simulink model "VMC_Integration"  (R2024a)
settings: Solver=FixedStepDiscrete  StartTime=0.0  StopTime=10.0  FixedStep=0.005  RelTol=1e-3
undefined symbols (not defined in the file): Degree_To_Rad_Factor
libraries: simulink x24, slpidlib x5
(part 1 of 3)
settings Model: Creator=Technic  LastModifiedBy=Technic
settings SolverCC: ZeroCrossControl=EnableAll
settings OptimizationCC: DefaultParameterBehavior=Inlined  DefaultUnderspecifiedDataType=single  EnhancedBackFolding=on  PassReuseOutputArgsAs=Individual arguments  ZeroExternalMemoryAtStartup=off  ZeroInternalMemoryAtStartup=off  OptimizeBlockOrder=speed  DifferentSizesBufferReuse=on  OptimizationCustomize=off  EfficientTunableParamExpr=on
settings DebuggingCC: AlgebraicLoopMsg=error  BlockPriorityViolationMsg=error  SolverPrmCheckMsg=error  ParameterPrecisionLossMsg=none  ParamPrecisionLossAbsoluteDiffThreshold=1e-12  ParamPrecisionLossRelativeDiffThreshold=1e-10  ParameterTunabilityLossMsg=error  UnnecessaryDatatypeConvMsg=warning  StateNameClashWarn=warning  AllowedUnitSystems=SI,SI (extended)  AllowAutomaticUnitConversions=off
settings HardwareCC: ProdBitPerPointer=32  ProdBitPerSizeT=32  ProdBitPerPtrDiffT=32  ProdLargestAtomicInteger=Long  ProdLargestAtomicFloat=Double  ProdWordSize=32  ProdHWDeviceType=NXP->Cortex-M4
settings SFSimCC: MATLABDynamicMemAlloc=off
settings RTWCC: Description=Embedded Coder  SystemTargetFile=ert.tlc  GenCodeOnly=on  TemplateMakefile=ert_default_tmf  GenerateReport=on  LaunchReport=on
settings CodeAppCC: ForceParamTrailComments=on  IgnoreCustomStorageClasses=off  OperatorAnnotations=on  SimulinkDataObjDesc=on  SFDataObjDesc=on  InsertBlockDesc=on
settings ERTTargetCC: TargetLangStandard=C99 (ISO)  GenerateSampleERTMain=on  InlinedParameterPlacement=NonHierarchical  ERTCustomFileTemplate=example_file_process.tlc

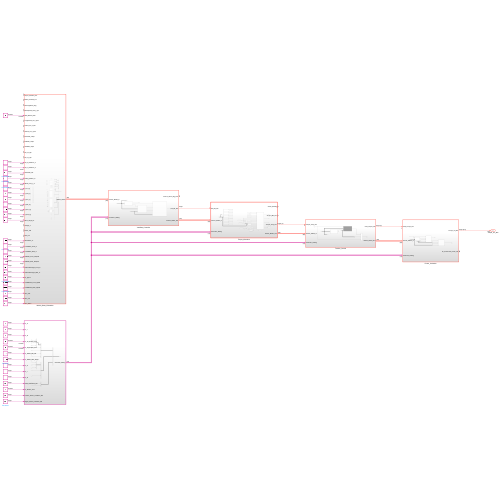
[thumbnail: Simulink's stored preview of the top-level diagram]
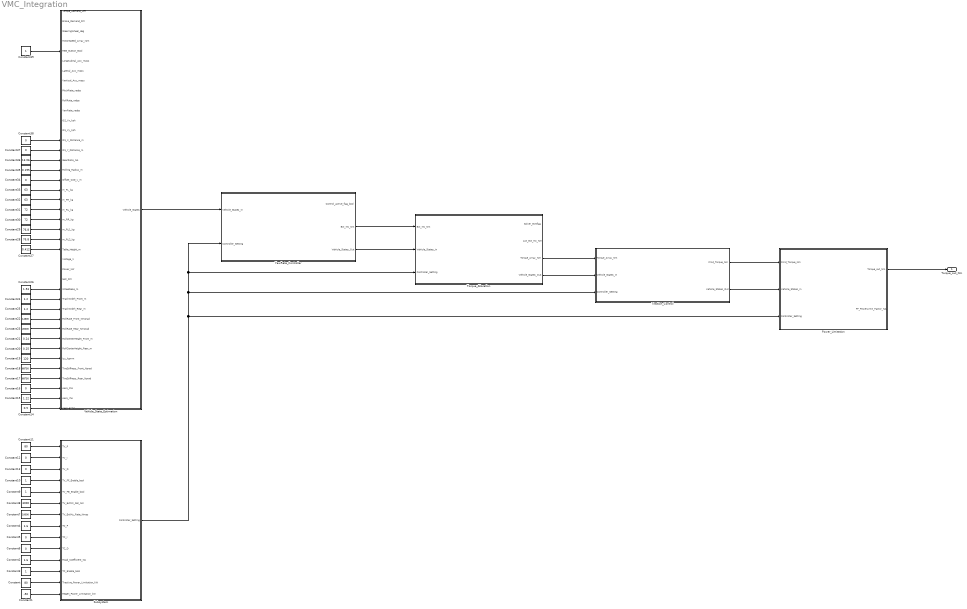
== system VMC_Integration ==
  Constant : Constant  Value=80  OutDataTypeStr=single
  Constant1 : Constant  Value=-50  OutDataTypeStr=single
  Constant{3,9..10,39} (4 alike) : Constant  OutDataTypeStr=boolean
  Constant11 : Constant  Value=80  OutDataTypeStr=single
  Constant{5..6,12..13,16,34,37..38} (8 alike) : Constant  Value=0  OutDataTypeStr=single
  Constant14 : Constant  Value=0.5  OutDataTypeStr=single
  Constant15 : Constant  Value=1.22  OutDataTypeStr=single
  Constant17 : Constant  Value=68750  OutDataTypeStr=single
  Constant18 : Constant  Value=68750  OutDataTypeStr=single
  Constant19 : Constant  Value=120  OutDataTypeStr=single
  Constant2 : Constant  Value=1.6  OutDataTypeStr=single
  Constant20 : Constant  Value=0.25  OutDataTypeStr=single
  Constant21 : Constant  Value=0.24  OutDataTypeStr=single
  Constant22 : Constant  Value=14600  OutDataTypeStr=single
  Constant23 : Constant  Value=45000  OutDataTypeStr=single
  Constant24 : Constant  Value=1.2  OutDataTypeStr=single
  Constant25 : Constant  Value=1.2  OutDataTypeStr=single
  Constant26 : Constant  Value=1.53  OutDataTypeStr=single
  Constant27 : Constant  Value=0.412  OutDataTypeStr=single
  Constant28 : Constant  Value=76.8  OutDataTypeStr=single
  Constant29 : Constant  Value=76.8  OutDataTypeStr=single
  Constant30 : Constant  Value=72  OutDataTypeStr=single
  Constant31 : Constant  Value=72  OutDataTypeStr=single
  Constant32 : Constant  Value=63  OutDataTypeStr=single
  Constant33 : Constant  Value=63  OutDataTypeStr=single
  Constant35 : Constant  Value=0.195  OutDataTypeStr=single
  Constant36 : Constant  Value=13.06  OutDataTypeStr=single
  Constant4 : Constant  Value=1.6  OutDataTypeStr=single
  Constant7 : Constant  Value=10000  OutDataTypeStr=single
  Constant8 : Constant  Value=3000  OutDataTypeStr=single
  Power_Limitation : Subsystem
  Subsystem : Subsystem
  Torque_Allocation : Subsystem  TreatAsAtomicUnit=on  RTWFcnName=Torque_Allocation
      settings: RTWSystemCode=Nonreusable function  RTWFcnNameOpts=User specified
  Traction_Control : Subsystem
  Vehicle_State_Estimation : Subsystem
  YawRate_Controller : Subsystem
  Torque_out_Nm : Outport
  wires:
  Vehicle_State_Estimation/1(Vehicle_States) -> YawRate_Controller/1(Vehicle_States_In)
  Subsystem/1(Controller_Setting) -> Torque_Allocation/3(Controller_Setting), YawRate_Controller/2(Controller_Setting), Traction_Control/3(Controller_Setting), Power_Limitation/3(Controller_Setting)
  YawRate_Controller/2(Ext_Mz_Nm) -> Torque_Allocation/1(Ext_Mz_Nm)
  YawRate_Controller/3(Vehicle_States_Out) -> Torque_Allocation/2(Vehicle_States_In)
  Torque_Allocation/3(Torque_Array_Nm) -> Traction_Control/1(Torque_Array_Nm)
  Traction_Control/2(Vehicle_States_Out) -> Power_Limitation/2(Vehicle_States_In)
  Traction_Control/1(Cmd_Torque_Nm) -> Power_Limitation/1(Cmd_Torque_Nm)
  Constant/1 -> Subsystem/13(Tractive_Power_Limitation_kW)
  Constant1/1 -> Subsystem/14(Regen_Power_Limitation_kW)
  Torque_Allocation/4(Vehicle_States_Out) -> Traction_Control/2(Vehicle_States_In)
  Power_Limitation/1(Torque_out_Nm) -> Torque_out_Nm/1
  Constant2/1 -> Subsystem/11(Road_Coefficient_NA)
  Constant3/1 -> Subsystem/12(TC_Enable_bool)
  Constant4/1 -> Subsystem/8(TC_P)
  Constant5/1 -> Subsystem/9(TC_I)
  Constant6/1 -> Subsystem/10(TC_D)
  Constant7/1 -> Subsystem/7(TV_ExtMz_Rate_Nmps)
  Constant8/1 -> Subsystem/6(TV_ExtMz_Sat_Nm)
  Constant9/1 -> Subsystem/5(TV_FB_Enable_bool)
  Constant10/1 -> Subsystem/4(TV_FF_Enable_bool)
  Constant11/1 -> Subsystem/1(TV_P)
  Constant12/1 -> Subsystem/2(TV_I)
  Constant13/1 -> Subsystem/3(TV_D)
  Constant14/1 -> Vehicle_State_Estimation/41(Aero_Ratio)
  Constant15/1 -> Vehicle_State_Estimation/40(Aero_rho)
  Constant16/1 -> Vehicle_State_Estimation/39(Aero_ClA)
  Constant17/1 -> Vehicle_State_Estimation/38(TireStiffness_Rear_Nprad)
  Constant18/1 -> Vehicle_State_Estimation/37(TireStiffness_Front_Nprad)
  Constant19/1 -> Vehicle_State_Estimation/36(Izz_kgmm)
  Constant20/1 -> Vehicle_State_Estimation/35(RollCenterHeight_Rear_m)
  Constant21/1 -> Vehicle_State_Estimation/34(RollCenterHeight_Front_m)
  Constant22/1 -> Vehicle_State_Estimation/32(RollRate_Front_Nmprad)
  Constant23/1 -> Vehicle_State_Estimation/33(RollRate_Rear_Nmprad)
  Constant24/1 -> Vehicle_State_Estimation/30(TrackWidth_Front_m)
  Constant25/1 -> Vehicle_State_Estimation/31(TrackWidth_Rear_m)
  Constant26/1 -> Vehicle_State_Estimation/29(Wheelbase_m)
  Constant27/1 -> Vehicle_State_Estimation/25(Table_Height_m)
  Constant28/1 -> Vehicle_State_Estimation/24(m_RL2_kg)
  Constant29/1 -> Vehicle_State_Estimation/23(m_RL1_kg)
  Constant30/1 -> Vehicle_State_Estimation/22(m_RR_kg)
  Constant31/1 -> Vehicle_State_Estimation/21(m_RL_kg)
  Constant32/1 -> Vehicle_State_Estimation/20(m_FR_kg)
  Constant33/1 -> Vehicle_State_Estimation/19(m_FL_kg)
  Constant34/1 -> Vehicle_State_Estimation/18(Offset_CoG_y_m)
  Constant35/1 -> Vehicle_State_Estimation/17(Rolling_Radius_m)
  Constant36/1 -> Vehicle_State_Estimation/16(GearRatio_NA)
  Constant37/1 -> Vehicle_State_Estimation/15(OS_Y_Distance_m)
  Constant38/1 -> Vehicle_State_Estimation/14(OS_X_Distance_m)
  Constant39/1 -> Vehicle_State_Estimation/5(REG_Button_Bool)

== system VMC_Integration/Power_Limitation ==
  Cmd_Torque_Nm : Inport
  Vehicle_States_In : Inport  Port=2
  Controller_Setting : Inport  Port=3
  Bus Selector : BusSelector  OutputSignals=Power_Limitation.Tractive_Power_Limitation_kW,Power_Limitation.Regen_Power_Limitation_kW
  Bus Selector1 : BusSelector  OutputSignals=Power_Limitation.Tractive_Power_Limitation_kW,Power_Limitation.Regen_Power_Limitation_kW
  Bus Selector2 : BusSelector  OutputSignals=Accumulator.Power_kW
  FeedForward_PowerLimit : MATLAB Function  TreatAsAtomicUnit=on
  MATLAB Function : MATLAB Function  TreatAsAtomicUnit=on
  Power_Estimation : Subsystem
  Torque_out_Nm : Outport
  FF_PowerLimit_Factor_NA : Outport  Port=2
  wires:
  Vehicle_States_In/1 -> Bus Selector2/1, Power_Estimation/2(Vehicle_States_In)
  Cmd_Torque_Nm/1 -> Power_Estimation/1(Cmd_Torque_Nm), FeedForward_PowerLimit/1(Torque)
  Controller_Setting/1 -> Bus Selector1/1, Bus Selector/1
  Bus Selector/1 -> FeedForward_PowerLimit/3(Tractive_Limit_Power)  "<Tractive_Power_Limitation_kW>"
  Power_Estimation/1(Est_Power_kW) -> FeedForward_PowerLimit/2(Est_Power)
  Bus Selector/2 -> FeedForward_PowerLimit/4(Regen_Limit_Power)  "<Regen_Power_Limitation_kW>"
  FeedForward_PowerLimit/2(Torque_out) -> MATLAB Function/1(Torque)
  Bus Selector1/1 -> MATLAB Function/2(Tractive_Limit_Power)  "<Tractive_Power_Limitation_kW>"
  Bus Selector1/2 -> MATLAB Function/3(Regen_Limit_Power)  "<Regen_Power_Limitation_kW>"
  Bus Selector2/1 -> MATLAB Function/4(Act_Power)  "<Power_kW>"
  MATLAB Function/1(Torque_out) -> Torque_out_Nm/1
  FeedForward_PowerLimit/1(factor) -> FF_PowerLimit_Factor_NA/1

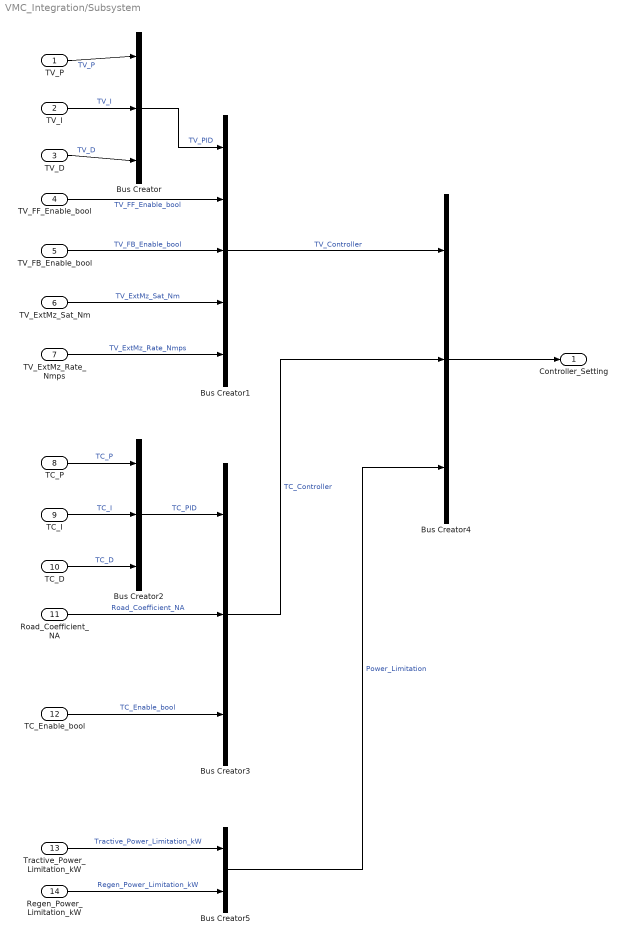
== system VMC_Integration/Subsystem ==
  TV_P : Inport
  TV_I : Inport  Port=2
  TV_D : Inport  Port=3
  TV_FF_Enable_bool : Inport  Port=4  OutDataTypeStr=boolean
  TV_FB_Enable_bool : Inport  Port=5  OutDataTypeStr=boolean
  TV_ExtMz_Sat_Nm : Inport  Port=6
  TV_ExtMz_Rate_Nmps : Inport  Port=7
  TC_P : Inport  Port=8
  TC_I : Inport  Port=9
  TC_D : Inport  Port=10
  Road_Coefficient_NA : Inport  Port=11
  TC_Enable_bool : Inport  Port=12
  Tractive_Power_Limitation_kW : Inport  Port=13
  Regen_Power_Limitation_kW : Inport  Port=14
  Bus Creator{,2..4} (4 alike) : BusCreator  Inputs=3
  Bus Creator1 : BusCreator  Inputs=5
  Bus Creator5 : BusCreator  Inputs=2
  Controller_Setting : Outport
  wires:
  TV_P/1 -> Bus Creator/1  "TV_P"
  TV_I/1 -> Bus Creator/2  "TV_I"
  TV_D/1 -> Bus Creator/3  "TV_D"
  Bus Creator/1 -> Bus Creator1/1  "TV_PID"
  TV_FF_Enable_bool/1 -> Bus Creator1/2  "TV_FF_Enable_bool"
  TV_FB_Enable_bool/1 -> Bus Creator1/3  "TV_FB_Enable_bool"
  TV_ExtMz_Sat_Nm/1 -> Bus Creator1/4  "TV_ExtMz_Sat_Nm"
  TV_ExtMz_Rate_Nmps/1 -> Bus Creator1/5  "TV_ExtMz_Rate_Nmps"
  TC_P/1 -> Bus Creator2/1  "TC_P"
  TC_I/1 -> Bus Creator2/2  "TC_I"
  TC_D/1 -> Bus Creator2/3  "TC_D"
  Bus Creator2/1 -> Bus Creator3/1  "TC_PID"
  Bus Creator1/1 -> Bus Creator4/1  "TV_Controller"
  Bus Creator3/1 -> Bus Creator4/2  "TC_Controller"
  Bus Creator4/1 -> Controller_Setting/1
  Road_Coefficient_NA/1 -> Bus Creator3/2  "Road_Coefficient_NA"
  TC_Enable_bool/1 -> Bus Creator3/3  "TC_Enable_bool"
  Bus Creator5/1 -> Bus Creator4/3  "Power_Limitation"
  Tractive_Power_Limitation_kW/1 -> Bus Creator5/1  "Tractive_Power_Limitation_kW"
  Regen_Power_Limitation_kW/1 -> Bus Creator5/2  "Regen_Power_Limitation_kW"

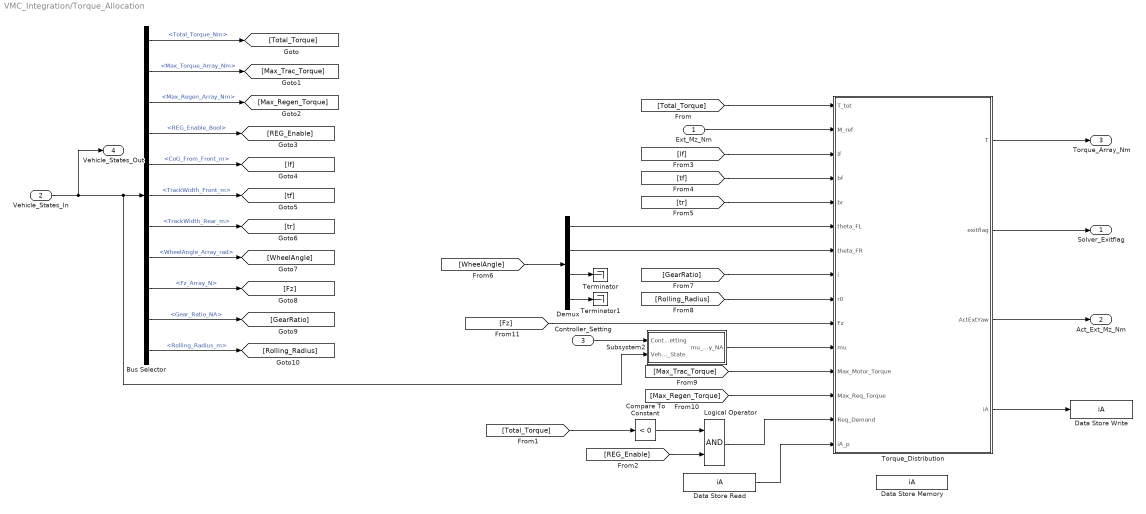
== system VMC_Integration/Torque_Allocation ==
  Ext_Mz_Nm : Inport
  Vehicle_States_In : Inport  Port=2
  Controller_Setting : Inport  Port=3
  Bus Selector : BusSelector  OutputSignals=Torque_Demand.Total_Torque_Nm,Torque_Demand.Max_Torque_Array_Nm,Torque_Demand.Max_Regen_Array_Nm,Torque_Demand.REG_Enable_Bool,Vehicle_Static_Parameter.CoG_From_Front_m,Vehicle_Static_Parameter.TrackWidth_Front_m,Vehicle_Static_Parameter.TrackWidth_Rear_m,WheelAngle.WheelAngle_Array_rad,Tire_Force.Fz_Array_N,Vehicle_Static_Parameter.Gear_Ratio_NA,Vehicle_Static_Parameter.Rolling_Radius_m
  Compare To Constant : simulink/Logic and Bit Operations/Compare To Constant  relop=<  const=0  OutDataTypeStr=boolean
  Data Store Memory : DataStoreMemory  DataStoreName=iA  WriteAfterWriteMsg=warning  InitialValue=[0,0,0,0,0,0,0,0]  ShowAdditionalParam=off  OutDataTypeStr=boolean
  Data Store Read : DataStoreRead  DataStoreName=iA  IndexOptions=Index vector (dialog)  Indices=1  OutputSizes=1
  Data Store Write : DataStoreWrite  DataStoreName=iA  IndexOptions=Index vector (dialog)  Indices=1  OutputSizes=1
  Demux : Demux
  Logical Operator : Logic  AllPortsSameDT=off  OutDataTypeStr=boolean
  Subsystem2 : Subsystem
  Terminator : Terminator
  Terminator1 : Terminator
  Torque_Distribution : MATLAB Function  TreatAsAtomicUnit=on
  Solver_Exitflag : Outport
  Act_Ext_Mz_Nm : Outport  Port=2
  Torque_Array_Nm : Outport  Port=3
  Vehicle_States_Out : Outport  Port=4
  wires:
  [Rolling_Radius] -> Torque_Distribution/9(r0)
  [tr] -> Torque_Distribution/5(br)
  [GearRatio] -> Torque_Distribution/8(i)
  [tf] -> Torque_Distribution/4(bf)
  [lf] -> Torque_Distribution/3(lf)
  [Max_Regen_Torque] -> Torque_Distribution/13(Max_Req_Torque)
  Torque_Distribution/2(exitflag) -> Solver_Exitflag/1
  Demux/1 -> Torque_Distribution/6(theta_FL)
  Demux/2 -> Torque_Distribution/7(theta_FR)
  [Fz] -> Torque_Distribution/10(Fz)
  [Max_Trac_Torque] -> Torque_Distribution/12(Max_Motor_Torque)
  Torque_Distribution/4(iA) -> Data Store Write/1
  Torque_Distribution/1(T) -> Torque_Array_Nm/1
  Data Store Read/1 -> Torque_Distribution/15(iA_p)
  Ext_Mz_Nm/1 -> Torque_Distribution/2(M_ref)
  Subsystem2/1(mu_x_Array_NA) -> Torque_Distribution/11(mu)
  Torque_Distribution/3(ActExtYaw) -> Act_Ext_Mz_Nm/1
  Logical Operator/1 -> Torque_Distribution/14(Req_Demand)
  Compare To Constant/1 -> Logical Operator/1
  [REG_Enable] -> Logical Operator/2
  Vehicle_States_In/1 -> Vehicle_States_Out/1, Subsystem2/2(Vehicle_State), Bus Selector/1
  Bus Selector/1 -> [Total_Torque]  "<Total_Torque_Nm>"
  Bus Selector/2 -> [Max_Trac_Torque]  "<Max_Torque_Array_Nm>"
  Bus Selector/3 -> [Max_Regen_Torque]  "<Max_Regen_Array_Nm>"
  Bus Selector/4 -> [REG_Enable]  "<REG_Enable_Bool>"
  Bus Selector/5 -> [lf]  "<CoG_From_Front_m>"
  Bus Selector/6 -> [tf]  "<TrackWidth_Front_m>"
  Bus Selector/7 -> [tr]  "<TrackWidth_Rear_m>"
  Bus Selector/8 -> [WheelAngle]  "<WheelAngle_Array_rad>"
  Bus Selector/9 -> [Fz]  "<Fz_Array_N>"
  Bus Selector/10 -> [GearRatio]  "<Gear_Ratio_NA>"
  Bus Selector/11 -> [Rolling_Radius]  "<Rolling_Radius_m>"
  [Total_Torque] -> Torque_Distribution/1(T_tot)
  [Total_Torque] -> Compare To Constant/1
  [WheelAngle] -> Demux/1
  Demux/3 -> Terminator/1
  Demux/4 -> Terminator1/1
  Controller_Setting/1 -> Subsystem2/1(Controller_Setting)

== system VMC_Integration/Traction_Control ==
  Torque_Array_Nm : Inport
  Vehicle_States_In : Inport  Port=2
  Controller_Setting : Inport  Port=3
  Bus Selector : BusSelector  OutputSignals=TC_Controller.TC_Enable_bool
  LSD_Enable : Subsystem
  LimitedSlipDifferential : Subsystem  Priority=2  TreatAsAtomicUnit=on  RTWFcnName=LimitedSlipDifferential
      settings: RTWSystemCode=Nonreusable function  RTWFcnNameOpts=User specified
  Switch : Switch  Criteria=u2 > Threshold  SaturateOnIntegerOverflow=off  InputSameDT=off
  Cmd_Torque_Nm : Outport
  Vehicle_States_Out : Outport  Port=2
  wires:
  Vehicle_States_In/1 -> Vehicle_States_Out/1, LimitedSlipDifferential/2(Vehicle_States), LSD_Enable/1(Vehicle_States)
  Controller_Setting/1 -> Bus Selector/1, LimitedSlipDifferential/4(Controller_Setting)
  LSD_Enable/1(LSD_Enable) -> LimitedSlipDifferential/3(LSD_Enable)
  Torque_Array_Nm/1 -> Switch/3, LimitedSlipDifferential/1(Cmd_Torque_Nm)
  Switch/1 -> Cmd_Torque_Nm/1
  LimitedSlipDifferential/1(LSD_Trq) -> Switch/1  "LSD_Trq"
  Bus Selector/1 -> Switch/2  "<TC_Enable_bool>"

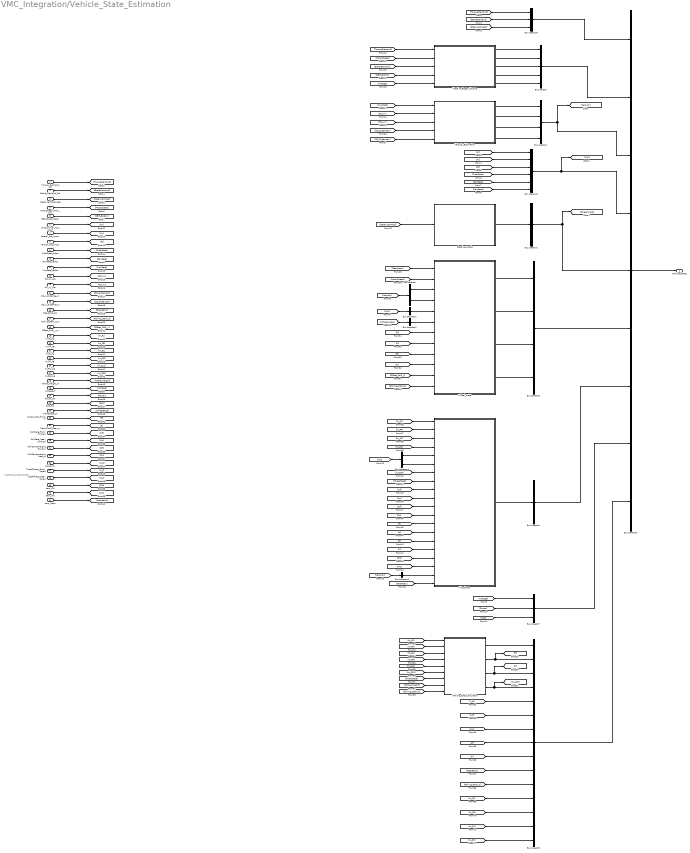
== system VMC_Integration/Vehicle_State_Estimation ==
  note: TireStiffness包含左右轮胎
  Torque_Demand_Pct : Inport  OutDataTypeStr=single
  Brake_Demand_Pct : Inport  Port=2  OutDataTypeStr=single
  SteeringWheel_deg : Inport  Port=3  OutDataTypeStr=single
  MotorSpeed_Array_rpm : Inport  Port=4  OutDataTypeStr=single
  REG_Button_Bool : Inport  Port=5  OutDataTypeStr=boolean
  Longitudinal_Acc_mpss : Inport  Port=6  OutDataTypeStr=single
  Lateral_Acc_mpss : Inport  Port=7  OutDataTypeStr=single
  Vertical_Acc_mpss : Inport  Port=8  OutDataTypeStr=single
  PitchRate_radps : Inport  Port=9  OutDataTypeStr=single
  RollRate_radps : Inport  Port=10  OutDataTypeStr=single
  YawRate_radps : Inport  Port=11  OutDataTypeStr=single
  OS_Vx_kph : Inport  Port=12  OutDataTypeStr=single
  OS_Vy_kph : Inport  Port=13  OutDataTypeStr=single
  OS_X_Distance_m : Inport  Port=14  OutDataTypeStr=single
  OS_Y_Distance_m : Inport  Port=15  OutDataTypeStr=single
  GearRatio_NA : Inport  Port=16  OutDataTypeStr=single
  Rolling_Radius_m : Inport  Port=17  OutDataTypeStr=single
  Offset_CoG_y_m : Inport  Port=18  OutDataTypeStr=single
  m_FL_kg : Inport  Port=19  OutDataTypeStr=single
  m_FR_kg : Inport  Port=20  OutDataTypeStr=single
  m_RL_kg : Inport  Port=21  OutDataTypeStr=single
  m_RR_kg : Inport  Port=22  OutDataTypeStr=single
  m_RL1_kg : Inport  Port=23  OutDataTypeStr=single
  m_RL2_kg : Inport  Port=24  OutDataTypeStr=single
  Table_Height_m : Inport  Port=25  OutDataTypeStr=single
  Voltage_V : Inport  Port=26  OutDataTypeStr=single
  Power_kW : Inport  Port=27  OutDataTypeStr=single
  SoC_Pct : Inport  Port=28  OutDataTypeStr=single
  Wheelbase_m : Inport  Port=29  OutDataTypeStr=single
  TrackWidth_Front_m : Inport  Port=30  OutDataTypeStr=single
  TrackWidth_Rear_m : Inport  Port=31  OutDataTypeStr=single
  RollRate_Front_Nmprad : Inport  Port=32  OutDataTypeStr=single
  RollRate_Rear_Nmprad : Inport  Port=33  OutDataTypeStr=single
  RollCenterHeight_Front_m : Inport  Port=34
  RollCenterHeight_Rear_m : Inport  Port=35
  Izz_kgmm : Inport  Port=36
  TireStiffness_Front_Nprad : Inport  Port=37
  TireStiffness_Rear_Nprad : Inport  Port=38
  Aero_ClA : Inport  Port=39
  Aero_rho : Inport  Port=40
  Aero_Ratio : Inport  Port=41
  Bus Creator : BusCreator  Inputs=5
  Bus Creator1 : BusCreator  Inputs=4
  Bus Creator2 : BusCreator  Inputs=1
  Bus Creator3 : BusCreator  Inputs=4
  Bus Creator4 : BusCreator  Inputs=1
  Bus Creator5 : BusCreator  Inputs=3
  Bus Creator6 : BusCreator  Inputs=6
  Bus Creator7 : BusCreator  Inputs=3
  Bus Creator8 : BusCreator  Inputs=9
  Bus Creator9 : BusCreator  Inputs=15
  Bus Selector : BusSelector  OutputSignals=CoG_Vx_mps,CoG_Vy_mps
  Bus Selector1 : BusSelector  OutputSignals=YawRate_radps
  Bus Selector2 : BusSelector  OutputSignals=WheelAngle_Array_rad
  Bus Selector3 : BusSelector  OutputSignals=CoG_V_mps
  Bus Selector4 : BusSelector  OutputSignals=Longitudinal_Acc_mpss,Lateral_Acc_mpss
  Steering_Angle : Subsystem
  Tire_Force : Subsystem
  Tractive_Regen_Torque : Subsystem
  Vehicle_CoG_Calculation : MATLAB Function  TreatAsAtomicUnit=on
  Velocity_Estimation : Subsystem
  Wheel_State : Subsystem
  Vehicle_States : Outport
  wires:
  Tractive_Regen_Torque/1(Total_Torque_Nm) -> Bus Creator/1  "Total_Torque_Nm"
  Tractive_Regen_Torque/2(Max_Torque_Array_Nm) -> Bus Creator/2  "Max_Torque_Array_Nm"
  Tractive_Regen_Torque/3(Max_Regen_Array_Nm) -> Bus Creator/3  "Max_Regen_Array_Nm"
  Velocity_Estimation/1(CoG_Vx_mps) -> Bus Creator1/1  "CoG_Vx_mps"
  Velocity_Estimation/2(CoG_Vy_mps) -> Bus Creator1/2  "CoG_Vy_mps"
  Velocity_Estimation/3(CoG_V_mps) -> Bus Creator1/3  "CoG_V_mps"
  Velocity_Estimation/4(OS_V_mps) -> Bus Creator1/4  "OS_V_mps"
  Steering_Angle/1(WheelAngle_Array_rad) -> Bus Creator2/1  "WheelAngle_Array_rad"
  Wheel_State/1(Act_WheelSpeed_Array_radps) -> Bus Creator3/1  "Act_WheelSpeed_Array_radps"
  Wheel_State/2(Ref_WheelSpeed_Array_radps) -> Bus Creator3/2  "Ref_WheelSpeed_Array_radps"
  Wheel_State/3(SlipRatio_Array_NA) -> Bus Creator3/3  "SlipRatio_Array_NA"
  Wheel_State/4(Tire_SlipAngle_Array_rad) -> Bus Creator3/4  "Tire_SlipAngle_Array_rad"
  Tire_Force/1(Fz_Array_N) -> Bus Creator4/1  "Fz_Array_N"
  [BrakeDemand] -> Bus Creator5/2  "Brake_Demand_Pct"
  [TorqueDemand] -> Bus Creator5/1  "Torque_Demand_Pct"
  Bus Creator5/1 -> Bus Creator8/1  "Driver_Demand"
  [SteeringWheel] -> Bus Creator5/3  "Steering_Demand_deg"
  Bus Creator/1 -> Bus Creator8/2  "Torque_Demand"
  [Ax] -> Bus Creator6/1  "Longitudinal_Acc_mpss"
  [Ay] -> Bus Creator6/2  "Lateral_Acc_mpss"
  [Az] -> Bus Creator6/3  "Vertical_Acc_mpss"
  [PitchRate] -> Bus Creator6/4  "PitchRate_radps"
  [RollRate] -> Bus Creator6/5  "RollRate_radps"
  [YawRate] -> Bus Creator6/6  "YawRate_radps"
  Bus Creator3/1 -> Bus Creator8/6  "Wheel"
  Bus Creator4/1 -> Bus Creator8/7  "Tire_Force"
  [Voltage] -> Bus Creator7/1  "Voltage_V"
  [Power] -> Bus Creator7/2  "Power_kW"
  [SoC] -> Bus Creator7/3  "SoC_Pct"
  Bus Creator7/1 -> Bus Creator8/8  "Accumulator"
  Bus Creator8/1 -> Vehicle_States/1
  [TorqueDemand] -> Tractive_Regen_Torque/1(Torque_Demand_Pct)
  [BrakeDemand] -> Tractive_Regen_Torque/3(Brake_Demand_Pct)
  [YawRate] -> Velocity_Estimation/1(IMU_YawRate_radps)
  [Voltage] -> Tractive_Regen_Torque/5(HV_Voltage_V)
  Bus Creator1/1 -> [Velocity], Bus Creator8/3  "Vehicle_Velocity"
  Bus Creator6/1 -> [IMU], Bus Creator8/4  "IMU"
  Bus Creator2/1 -> [WheelAngle], Bus Creator8/5  "WheelAngle"
  [Velocity] -> Bus Selector/1
  Bus Selector/1 -> Wheel_State/3(CoG_vx_mps)  "<CoG_Vx_mps>"
  Bus Selector/2 -> Wheel_State/4(CoG_vy_mps)  "<CoG_Vy_mps>"
  [IMU] -> Bus Selector1/1
  Bus Selector1/1 -> Wheel_State/5(Yawrate_radps)  "<YawRate_radps>"
  [WheelAngle] -> Bus Selector2/1
  Bus Selector2/1 -> Wheel_State/6(WheelAngle_Array_rad)  "<WheelAngle_Array_rad>"
  [Velocity] -> Bus Selector3/1
  Bus Selector3/1 -> Tire_Force/19(V_CoG_mps)  "<CoG_V_mps>"
  [IMU] -> Bus Selector4/1
  Bus Selector4/1 -> Tire_Force/5(ax_mpss)  "<Longitudinal_Acc_mpss>"
  Bus Selector4/2 -> Tire_Force/6(ay_mpss)  "<Lateral_Acc_mpss>"
  [SteeringWheel] -> Steering_Angle/1(SteeringWheelAngle_deg)
  [MotorSpeed] -> Tractive_Regen_Torque/2(MotorSpeed_Array_rpm)
  [REG_Button] -> Tractive_Regen_Torque/4(REG_Button_Bool)
  [OS_Vx] -> Velocity_Estimation/2(OS_Vx_kph)
  [OS_Vy] -> Velocity_Estimation/3(OS_Vy_kph)
  [OS_DistanceX] -> Velocity_Estimation/4(OS_X_Distance_m)
  [OS_DistanceY] -> Velocity_Estimation/5(OS_Y_Distance_m)
  [MotorSpeed] -> Wheel_State/2(MotorSpeed_Array_rpm)
  [GearRatio] -> Wheel_State/1(GearRatio_NA)
  [lf] -> Wheel_State/7(lf_m)
  [lr] -> Wheel_State/8(lr_m)
  [tf] -> Wheel_State/9(Trackwidth_Front_m)
  [tr] -> Wheel_State/10(Trackwidth_Rear_m)
  [Offset_CoG_y] -> Wheel_State/11(Offset_CoG_y_m)
  [Rolling_Radius] -> Wheel_State/12(Rolling_Radius_m)
  [m_FL] -> Tire_Force/1(m_FL_kg)
  [m_FR] -> Tire_Force/2(m_FR_kg)
  [m_RL] -> Tire_Force/3(m_RL_kg)
  [m_RR] -> Tire_Force/4(m_RR_kg)
  [h_CoG] -> Tire_Force/7(h_CoG_m)
  [WheelBase] -> Tire_Force/8(Wheelbase_m)
  [tf] -> Tire_Force/13(tf_m)
  [tr] -> Tire_Force/14(tr_m)
  [lf] -> Tire_Force/15(lf_m)
  [lr] -> Tire_Force/16(lr_m)
  [Zrr] -> Tire_Force/12(Zrr_m)
  [Zrf] -> Tire_Force/11(Zrf_m)
  [Krr] -> Tire_Force/10(Krr_Nmprad)
  [Krf] -> Tire_Force/9(Krf_Nmprad)
  [ClA] -> Tire_Force/17(ClA)
  [rho] -> Tire_Force/18(rho)
  [AeroRatio] -> Tire_Force/20(Aero_Ratio)
  Vehicle_CoG_Calculation/4(CoG_Height) -> [h_CoG], Bus Creator9/4  "CoG_Height"
  Vehicle_CoG_Calculation/2(CoG_From_Front) -> [lf], Bus Creator9/2  "CoG_From_Front_m"
  [m_RL1] -> Vehicle_CoG_Calculation/5(m_RL1)
  Vehicle_CoG_Calculation/3(CoG_From_Rear) -> [lr], Bus Creator9/3  "CoG_From_Rear_m"
  [m_FL] -> Vehicle_CoG_Calculation/1(m_FL)
  [Table_Height] -> Vehicle_CoG_Calculation/8(h)
  [Rolling_Radius] -> Vehicle_CoG_Calculation/9(r)
  [m_FR] -> Vehicle_CoG_Calculation/2(m_FR)
  Vehicle_CoG_Calculation/1(Overall_Mass) -> Bus Creator9/1  "Mass_kg"
  [m_RL] -> Vehicle_CoG_Calculation/3(m_RL)
  [WheelBase] -> Vehicle_CoG_Calculation/7(l)
  [m_RR] -> Vehicle_CoG_Calculation/4(m_RR)
  [m_RR1] -> Vehicle_CoG_Calculation/6(m_RR1)
  Bus Creator9/1 -> Bus Creator8/9  "Vehicle_Static_Parameter"
  Torque_Demand_Pct/1 -> [TorqueDemand]
  Brake_Demand_Pct/1 -> [BrakeDemand]
  SteeringWheel_deg/1 -> [SteeringWheel]
  MotorSpeed_Array_rpm/1 -> [MotorSpeed]
  REG_Button_Bool/1 -> [REG_Button]
  Longitudinal_Acc_mpss/1 -> [Ax]
  Lateral_Acc_mpss/1 -> [Ay]
  Vertical_Acc_mpss/1 -> [Az]
  PitchRate_radps/1 -> [PitchRate]
  RollRate_radps/1 -> [RollRate]
  YawRate_radps/1 -> [YawRate]
  OS_Vx_kph/1 -> [OS_Vx]
  OS_Vy_kph/1 -> [OS_Vy]
  OS_X_Distance_m/1 -> [OS_DistanceX]
  OS_Y_Distance_m/1 -> [OS_DistanceY]
  GearRatio_NA/1 -> [GearRatio]
  Rolling_Radius_m/1 -> [Rolling_Radius]
  Offset_CoG_y_m/1 -> [Offset_CoG_y]
  m_FL_kg/1 -> [m_FL]
  m_FR_kg/1 -> [m_FR]
  m_RL_kg/1 -> [m_RL]
  m_RR_kg/1 -> [m_RR]
  m_RL1_kg/1 -> [m_RL1]
  m_RL2_kg/1 -> [m_RR1]
  Table_Height_m/1 -> [Table_Height]
  Voltage_V/1 -> [Voltage]
  Power_kW/1 -> [Power]
  SoC_Pct/1 -> [SoC]
  Wheelbase_m/1 -> [WheelBase]
  TrackWidth_Front_m/1 -> [tf]
  TrackWidth_Rear_m/1 -> [tr]
  RollRate_Front_Nmprad/1 -> [Krf]
  RollRate_Rear_Nmprad/1 -> [Krr]
  RollCenterHeight_Front_m/1 -> [Zrf]
  RollCenterHeight_Rear_m/1 -> [Zrr]
  Aero_ClA/1 -> [ClA]
  Aero_rho/1 -> [rho]
  Aero_Ratio/1 -> [AeroRatio]
  [I_zz] -> Bus Creator9/5  "I_zz_kgmm"
  [K_f] -> Bus Creator9/6  "Kf_Nprad"
  [K_r] -> Bus Creator9/7  "Kr_Nprad"
  TireStiffness_Rear_Nprad/1 -> [K_r]
  TireStiffness_Front_Nprad/1 -> [K_f]
  Izz_kgmm/1 -> [I_zz]
  Tractive_Regen_Torque/4(REG_Enable_Bool) -> Bus Creator/4  "REG_Enable_Bool"
  [tf] -> Bus Creator9/8  "TrackWidth_Front_m"
  [tr] -> Bus Creator9/9  "TrackWidth_Rear_m"
  [GearRatio] -> Bus Creator9/10  "Gear_Ratio_NA"
  [Rolling_Radius] -> Bus Creator9/11  "Rolling_Radius_m"
  [m_FL] -> Bus Creator9/12  "m_FL_kg"
  [m_FR] -> Bus Creator9/13  "m_FR_kg"
  [m_RL] -> Bus Creator9/14  "m_RL_kg"
  [m_RR] -> Bus Creator9/15  "m_RR_kg"
  Tractive_Regen_Torque/5(MotorSpeed_Array_out_rpm) -> Bus Creator/5  "MotorSpeed_Array_rpm"

== system VMC_Integration/YawRate_Controller ==
  Vehicle_States_In : Inport
  Controller_Setting : Inport  Port=2
  CalMz_FB : Subsystem
  CalcMzDes_FF : Subsystem
  Subsystem : Subsystem
  Control_active_flag_bool : Outport
  Ext_Mz_Nm : Outport  Port=2
  Vehicle_States_Out : Outport  Port=3
  wires:
  Vehicle_States_In/1 -> Vehicle_States_Out/1, CalMz_FB/2(Vehicle_States), CalcMzDes_FF/1(Vehicle_States)
  CalcMzDes_FF/3(RefYawRate_radps) -> CalMz_FB/1(RefYawRate_radps)
  CalcMzDes_FF/1(Control_active_flag_bool) -> Control_active_flag_bool/1
  CalMz_FB/2(YawRateErr_radps) -> Subsystem/3(YawRateErr_radps)
  CalcMzDes_FF/2(ExtYawMoment_FF) -> Subsystem/1(ExtYawMoment_FF)
  CalMz_FB/1(ExtYawMoment_FB) -> Subsystem/2(ExtYawMoment_FB)
  Subsystem/1(Ext_Mz_Nm) -> Ext_Mz_Nm/1
  Controller_Setting/1 -> Subsystem/4(Controller_Setting), CalMz_FB/3(Controller_Setting)

== system VMC_Integration/Power_Limitation/Power_Estimation ==
  Cmd_Torque_Nm : Inport
  Vehicle_States_In : Inport  Port=2
  2-D Lookup Table : Lookup_n-D  BreakpointsForDimension1=[1.3,2.7,5.4,7.9,10.4,12.5,14.4,16,17.4,18.5,19.6]  BreakpointsForDimension2=[500,1000,2000,3000,4000,6000,10000,12000,16000,19000]  BreakpointsForDimension1DataTypeStr=single  BreakpointsForDimension2DataTypeStr=single  Table=reshape([64.37,58.42,44.94,35.59,29.14,24.17,20.41,17.31,14.82,12.81,11.17,71.33,70.84,60.81,51.9,44.78,38.71,33.76,29.4,25.75,22.67,20.05,73.64,77.57,73.35,67.02,61.01,52.22,50.04,45.1,40.67,36.72,33.21,74.7,80.4,78.82,74.26,69.41,64.39,59.65,54.87,50.41,46.3,42.51,75.43,82.01,81.94,78.54,74.57,70.24,65.99,61.55,57.28,53.25,49.44,76.57,83.92,85.43,83.42,80.62,77.3,73.88,70.1,66.34,62.67,59.09,77,85.16,88.2,87.58,85.93,83.73,81.33,78.56,75.7,72.77,69.82,77.08,85.44,88.88,88.65,87.34,85.48,83.42,80.97,78.4,75.75,73.06,77.56,85.97,89.71,89.94,88.86,87.37,85.66,83.56,81.34,79.02,76.63,78.14,86.5,90.44,90.86,90.16,88.98,87.59,85.81,83.91,81.91,79.83],11,10)  TableDataTypeStr=single  IntermediateResultsDataTypeStr=single  InternalRulePriority=Speed  OutDataTypeStr=single  RndMeth=Simplest  FractionDataTypeStr=single
      settings: InputPortMap=u0,u1
  Abs : Abs  SaturateOnIntegerOverflow=off
  Abs1 : Abs  SaturateOnIntegerOverflow=off
  Bus Selector : BusSelector  OutputSignals=Torque_Demand.MotorSpeed_Array_rpm
  MATLAB Function : MATLAB Function  TreatAsAtomicUnit=on
  Est_Power_kW : Outport
  wires:
  Cmd_Torque_Nm/1 -> MATLAB Function/1(Torque), Abs/1
  Abs/1 -> 2-D Lookup Table/1
  Abs1/1 -> 2-D Lookup Table/2
  Vehicle_States_In/1 -> Bus Selector/1
  Bus Selector/1 -> MATLAB Function/3(Speed), Abs1/1  "<MotorSpeed_Array_rpm>"
  2-D Lookup Table/1 -> MATLAB Function/2(Eta)
  MATLAB Function/1(Est_Power) -> Est_Power_kW/1

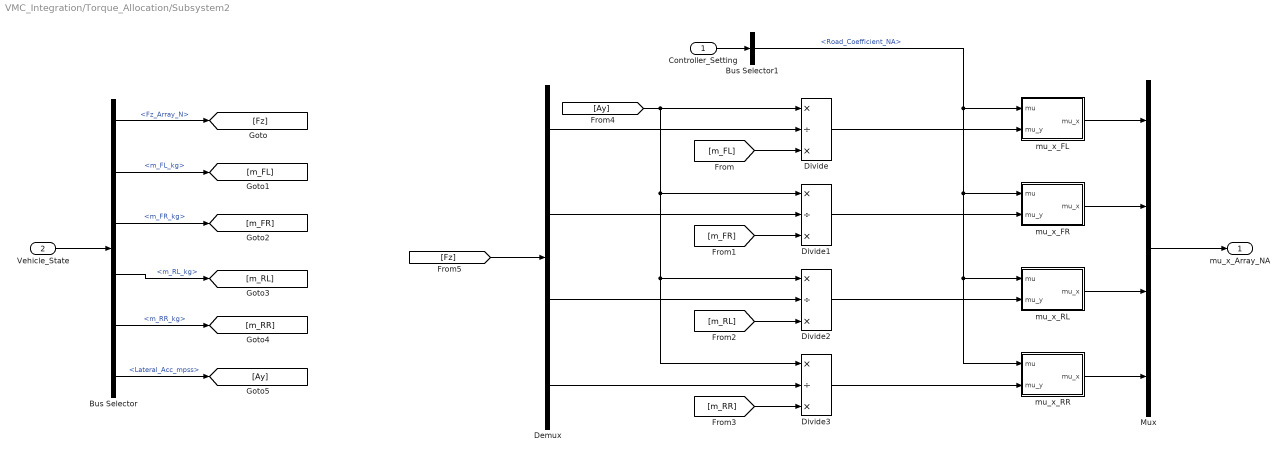
== system VMC_Integration/Torque_Allocation/Subsystem2 ==
  Controller_Setting : Inport
  Vehicle_State : Inport  Port=2
  Bus Selector : BusSelector  OutputSignals=Tire_Force.Fz_Array_N,Vehicle_Static_Parameter.m_FL_kg,Vehicle_Static_Parameter.m_FR_kg,Vehicle_Static_Parameter.m_RL_kg,Vehicle_Static_Parameter.m_RR_kg,IMU.Lateral_Acc_mpss
  Bus Selector1 : BusSelector  OutputSignals=TC_Controller.Road_Coefficient_NA
  Demux : Demux
  Divide{,1..3} (4 alike) : Product  Inputs=*/*  OutDataTypeStr=single
  Mux : Mux
  mu_x_FL : MATLAB Function  TreatAsAtomicUnit=on
  mu_x_FR : MATLAB Function  TreatAsAtomicUnit=on
  mu_x_RL : MATLAB Function  TreatAsAtomicUnit=on
  mu_x_RR : MATLAB Function  TreatAsAtomicUnit=on
  mu_x_Array_NA : Outport
  wires:
  [m_FL] -> Divide/3
  Vehicle_State/1 -> Bus Selector/1
  Demux/1 -> Divide/2
  Demux/2 -> Divide1/2
  Demux/3 -> Divide2/2
  Demux/4 -> Divide3/2
  [m_FR] -> Divide1/3
  [m_RL] -> Divide2/3
  [m_RR] -> Divide3/3
  Bus Selector1/1 -> mu_x_RR/1(mu), mu_x_RL/1(mu), mu_x_FR/1(mu), mu_x_FL/1(mu)  "<Road_Coefficient_NA>"
  Divide/1 -> mu_x_FL/2(mu_y)
  Divide1/1 -> mu_x_FR/2(mu_y)
  Divide2/1 -> mu_x_RL/2(mu_y)
  Divide3/1 -> mu_x_RR/2(mu_y)
  mu_x_FL/1(mu_x) -> Mux/1
  mu_x_FR/1(mu_x) -> Mux/2
  mu_x_RL/1(mu_x) -> Mux/3
  mu_x_RR/1(mu_x) -> Mux/4
  Mux/1 -> mu_x_Array_NA/1
  [Ay] -> Divide3/1, Divide2/1, Divide1/1, Divide/1
  Bus Selector/1 -> [Fz]  "<Fz_Array_N>"
  Bus Selector/2 -> [m_FL]  "<m_FL_kg>"
  Bus Selector/3 -> [m_FR]  "<m_FR_kg>"
  Bus Selector/4 -> [m_RL]  "<m_RL_kg>"
  Bus Selector/5 -> [m_RR]  "<m_RR_kg>"
  Bus Selector/6 -> [Ay]  "<Lateral_Acc_mpss>"
  [Fz] -> Demux/1
  Controller_Setting/1 -> Bus Selector1/1

== system VMC_Integration/Traction_Control/LSD_Enable ==
  Vehicle_States : Inport
  Bus Selector : BusSelector  OutputSignals=Driver_Demand.Brake_Demand_Pct,Wheel.Act_WheelSpeed_Array_radps,Wheel.SlipRatio_Array_NA
  Demux : Demux
  Demux1 : Demux
  LSD_EnableFL : Subsystem
  LSD_EnableFR : Subsystem
  LSD_EnableRL : Subsystem
  "LSD_EnableRR " : Subsystem
  Mux1 : Mux
  LSD_Enable : Outport
  wires:
  Demux/3 -> LSD_EnableRL/2(WhlSpdActlRL)
  "LSD_EnableRR "/1(LSD_EnableFL) -> Mux1/4  "LSD_EnableRR"
  Demux1/3 -> LSD_EnableRL/3(WhlSpdRefRL)
  Demux/2 -> LSD_EnableFR/2(WhlSpdActlFR)
  LSD_EnableRL/1(LSD_EnableFL) -> Mux1/3  "LSD_EnableRL"
  Demux/1 -> LSD_EnableFL/2(WhlSpdActlFL)
  Bus Selector/3 -> Demux1/1  "<SlipRatio_Array_NA>"
  LSD_EnableFR/1(LSD_EnableFL) -> Mux1/2  "LSD_EnableFR"
  Demux1/4 -> "LSD_EnableRR "/3(WhlSpdRefRR)
  Bus Selector/1 -> LSD_EnableFR/1(BrkDmd), "LSD_EnableRR "/1(BrkDmd), LSD_EnableRL/1(BrkDmd), LSD_EnableFL/1(BrkDmd)  "<Brake_Demand_Pct>"
  Demux1/2 -> LSD_EnableFR/3(WhlSpdRefFR)
  Demux/4 -> "LSD_EnableRR "/2(WhlSpdActlRR)
  Mux1/1 -> LSD_Enable/1  "LSD_Enable"
  Demux1/1 -> LSD_EnableFL/3(WhlSpdRefFL)
  LSD_EnableFL/1(LSD_EnableFL) -> Mux1/1  "LSD_EnableFL"
  Vehicle_States/1 -> Bus Selector/1
  Bus Selector/2 -> Demux/1  "<Act_WheelSpeed_Array_radps>"

== system VMC_Integration/Traction_Control/LimitedSlipDifferential ==
  Cmd_Torque_Nm : Inport
  Vehicle_States : Inport  Port=2
  LSD_Enable : Inport  Port=3
  Controller_Setting : Inport  Port=4
  Demux : Demux
  LSD_Ctrl : Subsystem
  Mux : Mux
  PID_CtrlFL : Subsystem
  PID_CtrlFR : Subsystem
  PID_CtrlRL : Subsystem
  PID_CtrlRR : Subsystem
  Subsystem : Subsystem
  LSD_Trq : Outport  VectorParamsAs1DForOutWhenUnconnected=off
  wires:
  PID_CtrlFL/1(LSD_TrqFL) -> Mux/1  "LSD_TrqFL"
  PID_CtrlRL/1(LSD_TrqRL) -> Mux/3  "LSD_TrqRL"
  PID_CtrlRR/1(LSD_TrqRR) -> Mux/4  "LSD_TrqRR"
  Cmd_Torque_Nm/1 -> Demux/1
  Demux/1 -> PID_CtrlFL/2(EDS_TrqFL)  "TrqFL"
  Demux/2 -> PID_CtrlFR/2(EDS_TrqFR)  "TrqFR"
  Demux/3 -> PID_CtrlRL/2(EDS_TrqRL)  "TrqRL"
  Demux/4 -> PID_CtrlRR/2(EDS_TrqRR)  "TrqRR"
  LSD_Ctrl/1(LSD_CtrlFL) -> PID_CtrlFL/1(LSD_CtrlFL)
  LSD_Ctrl/2(LSD_CtrlFR) -> PID_CtrlFR/1(LSD_CtrlFR)
  LSD_Ctrl/3(LSD_CtrlRL) -> PID_CtrlRL/1(LSD_CtrlRL)
  LSD_Ctrl/4(LSD_CtrlRR) -> PID_CtrlRR/1(LSD_CtrlRR)
  Mux/1 -> LSD_Trq/1  "LSD_Trq"
  PID_CtrlFR/1(LSD_TrqFR) -> Mux/2  "LSD_TrqFR"
  Vehicle_States/1 -> LSD_Ctrl/1(Vehicle_States)
  LSD_Enable/1 -> Subsystem/1(LSD_Enable), LSD_Ctrl/2(LSD_Enable)
  Controller_Setting/1 -> Subsystem/2(Controller_Setting)
  Subsystem/1(PID_Setting) -> PID_CtrlRR/3(PID_Setting), PID_CtrlRL/3(PID_Setting), PID_CtrlFR/3(PID_Setting), PID_CtrlFL/3(PID_Setting)

== system VMC_Integration/Vehicle_State_Estimation/Steering_Angle ==
  SteeringWheelAngle_deg : Inport
  Constant3 : Constant  Value=0  OutDataTypeStr=single  SampleTime=-1
  Constant4 : Constant  Value=0  OutDataTypeStr=single  SampleTime=-1
  FWA_FL_Table_deg : Lookup_n-D  NumberOfTableDimensions=1  BreakpointsForDimension1=|  BreakpointsForDimension1DataTypeStr=single  Table=|  TableDataTypeStr=single  IntermediateResultsDataTypeStr=single  InternalRulePriority=Speed  OutDataTypeStr=single  RndMeth=Simplest  FractionDataTypeStr=single
      BreakpointsForDimension1=|
      | [-117
      | -116
      | -115
      | -114
      | -113
      | -112
      | -111
      | -110
      | -109
      | -108
      | -107
      | -106
      | -105
      | -104
      | -103
      | -102
      | -101
      | -100
      | -99
      | -98
      | -97
      | -96
      | -95
      | -94
      | -93
      | -92
      | -91
      | -90
      | -89
      | -88
      | -87
      | -86
      | -85
      | -84
      | -83
      | -82
      | -81
      | -80
      | -79
      | -78
      | -77
      | -76
      | -75
      | -74
      | -73
      | -72
      | -71
      | -70
      | -69
      | -68
      | -67
      | -66
      | -65
      | -64
      | -63
      | -62
      | -61
      | -60
      | -59
      | -58
      | -57
      | -56
      | -55
      | -54
      | -53
      | -52
      | -51
      | -50
      | -49
      | -48
      | -47
      | -46
      | -45
      | -44
      | -43
      | -42
      | -41
      | -40
      | -39
      | -38
      | -37
      | -36
      | -35
      | -34
      | -33
      | -32
      | -31
      | -30
      | -29
      | -28
      | -27
      | -26
      | -25
      | -24
      | -23
      | -22
      | -21
      | -20
      | -19
      | -18
      | -17
      | -16
      | -15
      | -14
      | -13
      | -12
      | -11
      | -10
      | -9
      | -8
      | -7
      | -6
      | -5
      | -4
      | -3
      | -2
      | -1
      | 0
      | 1
      | 2
      | 3
      | 4
      | 5
      | 6
      | 7
      | 8
      | 9
      | 10
      | 11
      | 12
      | 13
      | 14
      | 15
      | 16
      | 17
      | 18
      | 19
      | 20
      | 21
      | 22
      | 23
      | 24
      | 25
      | 26
      | 27
      | 28
      | 29
      | 30
      | 31
      | 32
      | 33
      | 34
      | 35
      | 36
      | 37
      | 38
      | 39
      | 40
      | 41
      | 42
      | 43
      | 44
      | 45
      | 46
      | 47
      | 48
      | 49
      | 50
      | 51
      | 52
      | 53
      | 54
      | 55
      | 56
      | 57
      | 58
      | 59
      | 60
      | 61
      | 62
      | 63
      | 64
      | 65
      | 66
      | 67
      | 68
      | 69
      | 70
      | 71
      | 72
      | 73
      | 74
      | 75
      | 76
      | 77
      | 78
      | 79
      | 80
      | 81
      | 82
      | 83
      | 84
      | 85
      | 86
      | 87
      | 88
      | 89
      | 90
      | 91
      | 92
      | 93
      | 94
      | 95
      | 96
      | 97
      | 98
      | 99
      | 100
      | 101
      | 102
      | 103
      | 104
      | 105
      | 106
      | 107
      | 108
      | 109
      | 110
      | 111
      | 112
      | 113
      | 114
      | 115
      | 116
      | 117]
      Table=|
      | [-23.05316527
      | -22.85986982
      | -22.66659264
      | -22.47333151
      | -22.28008425
      | -22.08684866
      | -21.89362256
      | -21.70040379
      | -21.50719018
      | -21.31397955
      | -21.12076975
      | -20.92755864
      | -20.73434405
      | -20.54112386
      | -20.34789591
      | -20.15465809
      | -19.96140824
      | -19.76814426
      | -19.57486401
      | -19.38156538
      | -19.18824624
      | -18.99490448
      | -18.801538
      | -18.60814467
      | -18.4147224
      | -18.22126908
      | -18.0277826
      | -17.83426085
      | -17.64070175
      | -17.44710317
      | -17.25346304
      | -17.05977924
      | -16.86604968
      | -16.67227225
      | -16.47844486
      | -16.2845654
      | -16.09063178
      | -15.89664189
      | -15.70259363
      | -15.5084849
      | -15.31431358
      | -15.12007757
      | -14.92577477
      | -14.73140306
      | -14.53696032
      | -14.34244444
      | -14.14785329
      | -13.95318476
      | -13.75843671
      | -13.56360702
      | -13.36869356
      | -13.17369417
      | -12.97860673
      | -12.78342908
      | -12.58815908
      | -12.39279455
      | -12.19733335
      | -12.00177331
      | -11.80611224
      | -11.61034798
      | -11.41447833
      | -11.2185011
      | -11.0224141
      | -10.82621511
      | -10.62990193
      | -10.43347233
      | -10.23692409
      | -10.04025496
      | -9.843462713
      | -9.646545082
      | -9.449499809
      | -9.252324623
      | -9.055017243
      | -8.857575379
      | -8.659996732
      | -8.46227899
      | -8.264419833
      | -8.066416931
      | -7.868267939
      | -7.669970506
      | -7.471522265
      | -7.27292084
      | -7.07416384
      | -6.875248864
      | -6.676173498
      | -6.476935313
      | -6.277531868
      | -6.077960708
      | -5.878219363
      | -5.678305351
      | -5.478216172
      | -5.277949314
      | -5.077502247
      | -4.876872426
      | -4.676057291
      | -4.475054264
      | -4.273860752
      | -4.072474141
      | -3.870891803
      | -3.669111092
      | -3.467129341
      | -3.264943865
      | -3.062551963
      | -2.859950909
      | -2.657137961
      | -2.454110356
      | -2.250865308
      | -2.047400013
      | -1.843711642
      | -1.639797346
      | -1.435654252
      | -1.231279465
      | -1.026670065
      | -0.82182311
      | -0.616735632
      | -0.411404637
      | -0.205827108
      | 0
      | 0.206079759
      | 0.412415266
      | 0.619009648
      | 0.825866059
      | 1.032987682
      | 1.240377731
      | 1.448039447
      | 1.655976105
      | 1.864191008
      | 2.072687493
      | 2.28146893
      | 2.49053872
      | 2.6999003
      | 2.909557141
      | 3.119512748
      | 3.329770663
      | 3.540334465
      | 3.75120777
      | 3.962394233
      | 4.173897546
      | 4.385721443
      | 4.597869697
      | 4.810346123
      | 5.02315458
      | 5.236298967
      | 5.449783228
      | 5.663611355
      | 5.877787381
      | 6.09231539
      | 6.307199511
      | 6.522443924
      | 6.738052856
      | 6.954030589
      | 7.170381452
      | 7.387109832
      | 7.604220167
      | 7.821716951
      | 8.039604735
      | 8.257888127
      | 8.476571794
      | 8.695660466
      | 8.915158929
      | 9.135072038
      | 9.355404708
      | 9.576161921
      | 9.797348726
      | 10.01897024
      | 10.24103166
      | 10.46353823
      | 10.68649529
      | 10.90990825
      | 11.1337826
      | 11.35812389
      | 11.58293777
      | 11.80822996
      | 12.03400628
      | 12.26027261
      | 12.48703495
      | 12.71429936
      | 12.94207201
      | 13.17035916
      | 13.39916716
      | 13.62850247
      | 13.85837164
      | 14.08878133
      | 14.3197383
      | 14.55124944
      | 14.78332172
      | 15.01596225
      | 15.24917823
      | 15.48297702
      | 15.71736605
      | 15.95235293
      | 16.18794536
      | 16.42415119
      | 16.66097841
      | 16.89843513
      | 17.13652963
      | 17.3752703
      | 17.61466573
      | 17.85472462
      | 18.09545586
      | 18.33686848
      | 18.5789717
      | 18.82177488
      | 19.06528761
      | 19.3095196
      | 19.55448079
      | 19.80018131
      | 20.04663146
      | 20.29384178
      | 20.54182299
      | 20.79058604
      | 21.0401421
      | 21.29050257
      | 21.54167908
      | 21.79368351
      | 22.04652799
      | 22.3002249
      | 22.55478688
      | 22.81022687
      | 23.06655806
      | 23.32379396
      | 23.58194836
      | 23.84103537
      | 24.10106942
      | 24.36206527
      | 24.62403801
      | 24.88700311
      | 25.15097637
      | 25.415974
      | 25.68201259
      | 25.94910911
      | 26.217281
      | 26.48654607
      | 26.75692263
      | 27.02842943
      | ]
  FWA_FR_Table_deg : Lookup_n-D  NumberOfTableDimensions=1  BreakpointsForDimension1=|  BreakpointsForDimension1DataTypeStr=single  Table=|  TableDataTypeStr=single  IntermediateResultsDataTypeStr=single  InternalRulePriority=Speed  OutDataTypeStr=single  RndMeth=Simplest  FractionDataTypeStr=single
      BreakpointsForDimension1=|
      | [-117
      | -116
      | -115
      | -114
      | -113
      | -112
      | -111
      | -110
      | -109
      | -108
      | -107
      | -106
      | -105
      | -104
      | -103
      | -102
      | -101
      | -100
      | -99
      | -98
      | -97
      | -96
      | -95
      | -94
      | -93
      | -92
      | -91
      | -90
      | -89
      | -88
      | -87
      | -86
      | -85
      | -84
      | -83
      | -82
      | -81
      | -80
      | -79
      | -78
      | -77
      | -76
      | -75
      | -74
      | -73
      | -72
      | -71
      | -70
      | -69
      | -68
      | -67
      | -66
      | -65
      | -64
      | -63
      | -62
      | -61
      | -60
      | -59
      | -58
      | -57
      | -56
      | -55
      | -54
      | -53
      | -52
      | -51
      | -50
      | -49
      | -48
      | -47
      | -46
      | -45
      | -44
      | -43
      | -42
      | -41
      | -40
      | -39
      | -38
      | -37
      | -36
      | -35
      | -34
      | -33
      | -32
      | -31
      | -30
      | -29
      | -28
      | -27
      | -26
      | -25
      | -24
      | -23
      | -22
      | -21
      | -20
      | -19
      | -18
      | -17
      | -16
      | -15
      | -14
      | -13
      | -12
      | -11
      | -10
      | -9
      | -8
      | -7
      | -6
      | -5
      | -4
      | -3
      | -2
      | -1
      | 0
      | 1
      | 2
      | 3
      | 4
      | 5
      | 6
      | 7
      | 8
      | 9
      | 10
      | 11
      | 12
      | 13
      | 14
      | 15
      | 16
      | 17
      | 18
      | 19
      | 20
      | 21
      | 22
      | 23
      | 24
      | 25
      | 26
      | 27
      | 28
      | 29
      | 30
      | 31
      | 32
      | 33
      | 34
      | 35
      | 36
      | 37
      | 38
      | 39
      | 40
      | 41
      | 42
      | 43
      | 44
      | 45
      | 46
      | 47
      | 48
      | 49
      | 50
      | 51
      | 52
      | 53
      | 54
      | 55
      | 56
      | 57
      | 58
      | 59
      | 60
      | 61
      | 62
      | 63
      | 64
      | 65
      | 66
      | 67
      | 68
      | 69
      | 70
      | 71
      | 72
      | 73
      | 74
      | 75
      | 76
      | 77
      | 78
      | 79
      | 80
      | 81
      | 82
      | 83
      | 84
      | 85
      | 86
      | 87
      | 88
      | 89
      | 90
      | 91
      | 92
      | 93
      | 94
      | 95
      | 96
      | 97
      | 98
      | 99
      | 100
      | 101
      | 102
      | 103
      | 104
      | 105
      | 106
      | 107
      | 108
      | 109
      | 110
      | 111
      | 112
      | 113
      | 114
      | 115
      | 116
      | 117]
      Table=|
      | [-27.02842943
      | -26.75692263
      | -26.48654607
      | -26.217281
      | -25.94910911
      | -25.68201259
      | -25.415974
      | -25.15097637
      | -24.88700311
      | -24.62403801
      | -24.36206527
      | -24.10106942
      | -23.84103537
      | -23.58194836
      | -23.32379396
      | -23.06655806
      | -22.81022687
      | -22.55478688
      | -22.3002249
      | -22.04652799
      | -21.79368351
      | -21.54167908
      | -21.29050257
      | -21.0401421
      | -20.79058604
      | -20.54182299
      | -20.29384178
      | -20.04663146
      | -19.80018131
      | -19.55448079
      | -19.3095196
      | -19.06528761
      | -18.82177488
      | -18.5789717
      | -18.33686848
      | -18.09545586
      | -17.85472462
      | -17.61466573
      | -17.3752703
      | -17.13652963
      | -16.89843513
      | -16.66097841
      | -16.42415119
      | -16.18794536
      | -15.95235293
      | -15.71736605
      | -15.48297702
      | -15.24917823
      | -15.01596225
      | -14.78332172
      | -14.55124944
      | -14.3197383
      | -14.08878133
      | -13.85837164
      | -13.62850247
      | -13.39916716
      | -13.17035916
      | -12.94207201
      | -12.71429936
      | -12.48703495
      | -12.26027261
      | -12.03400628
      | -11.80822996
      | -11.58293777
      | -11.35812389
      | -11.1337826
      | -10.90990825
      | -10.68649529
      | -10.46353823
      | -10.24103166
      | -10.01897024
      | -9.797348726
      | -9.576161921
      | -9.355404708
      | -9.135072038
      | -8.915158929
      | -8.695660466
      | -8.476571794
      | -8.257888127
      | -8.039604735
      | -7.821716951
      | -7.604220167
      | -7.387109832
      | -7.170381452
      | -6.954030589
      | -6.738052856
      | -6.522443924
      | -6.307199511
      | -6.09231539
      | -5.877787381
      | -5.663611355
      | -5.449783228
      | -5.236298967
      | -5.02315458
      | -4.810346123
      | -4.597869697
      | -4.385721443
      | -4.173897546
      | -3.962394233
      | -3.75120777
      | -3.540334465
      | -3.329770663
      | -3.119512748
      | -2.909557141
      | -2.6999003
      | -2.49053872
      | -2.28146893
      | -2.072687493
      | -1.864191008
      | -1.655976105
      | -1.448039447
      | -1.240377731
      | -1.032987682
      | -0.825866059
      | -0.619009648
      | -0.412415266
      | -0.206079759
      | 0
      | 0.205827108
      | 0.411404637
      | 0.616735632
      | 0.82182311
      | 1.026670065
      | 1.231279465
      | 1.435654252
      | 1.639797346
      | 1.843711642
      | 2.047400013
      | 2.250865308
      | 2.454110356
      | 2.657137961
      | 2.859950909
      | 3.062551963
      | 3.264943865
      | 3.467129341
      | 3.669111092
      | 3.870891803
      | 4.072474141
      | 4.273860752
      | 4.475054264
      | 4.676057291
      | 4.876872426
      | 5.077502247
      | 5.277949314
      | 5.478216172
      | 5.678305351
      | 5.878219363
      | 6.077960708
      | 6.277531868
      | 6.476935313
      | 6.676173498
      | 6.875248864
      | 7.07416384
      | 7.27292084
      | 7.471522265
      | 7.669970506
      | 7.868267939
      | 8.066416931
      | 8.264419833
      | 8.46227899
      | 8.659996732
      | 8.857575379
      | 9.055017243
      | 9.252324623
      | 9.449499809
      | 9.646545082
      | 9.843462713
      | 10.04025496
      | 10.23692409
      | 10.43347233
      | 10.62990193
      | 10.82621511
      | 11.0224141
      | 11.2185011
      | 11.41447833
      | 11.61034798
      | 11.80611224
      | 12.00177331
      | 12.19733335
      | 12.39279455
      | 12.58815908
      | 12.78342908
      | 12.97860673
      | 13.17369417
      | 13.36869356
      | 13.56360702
      | 13.75843671
      | 13.95318476
      | 14.14785329
      | 14.34244444
      | 14.53696032
      | 14.73140306
      | 14.92577477
      | 15.12007757
      | 15.31431358
      | 15.5084849
      | 15.70259363
      | 15.89664189
      | 16.09063178
      | 16.2845654
      | 16.47844486
      | 16.67227225
      | 16.86604968
      | 17.05977924
      | 17.25346304
      | 17.44710317
      | 17.64070175
      | 17.83426085
      | 18.0277826
      | 18.22126908
      | 18.4147224
      | 18.60814467
      | 18.801538
      | 18.99490448
      | 19.18824624
      | 19.38156538
      | 19.57486401
      | 19.76814426
      | 19.96140824
      | 20.15465809
      | 20.34789591
      | 20.54112386
      | 20.73434405
      | 20.92755864
      | 21.12076975
      | 21.31397955
      | 21.50719018
      | 21.70040379
      | 21.89362256
      | 22.08684866
      | 22.28008425
      | 22.47333151
      | 22.66659264
      | 22.85986982
      | 23.05316527
      | ]
  Gain6 : Gain  Commented=through  Gain=Degree_To_Rad_Factor  OutDataTypeStr=single
  Gain7 : Gain  Commented=through  Gain=Degree_To_Rad_Factor  OutDataTypeStr=single
  Mux : Mux
  Saturation : Saturate  UpperLimit=117  LowerLimit=-117  OutDataTypeStr=single
  WheelAngle_Array_rad : Outport
  wires:
  FWA_FL_Table_deg/1 -> Gain6/1
  Gain6/1 -> Mux/1  "Steering_Angle_ByRad"
  Mux/1 -> WheelAngle_Array_rad/1
  Constant3/1 -> Mux/3  "RL_Wheel_Angle"
  FWA_FR_Table_deg/1 -> Gain7/1
  Gain7/1 -> Mux/2  "Steering_Angle_ByRad"
  Constant4/1 -> Mux/4  "RR_Wheel_Angle"
  Saturation/1 -> FWA_FR_Table_deg/1, FWA_FL_Table_deg/1
  SteeringWheelAngle_deg/1 -> Saturation/1
